simulink model "circuitosLogicos"  (R2014a)
settings: Solver=ode45  StartTime=0.0  StopTime=inf  MaxStep=0.01  RelTol=1e-3
settings Model: Creator=gbtom  LastModifiedBy=gbtom

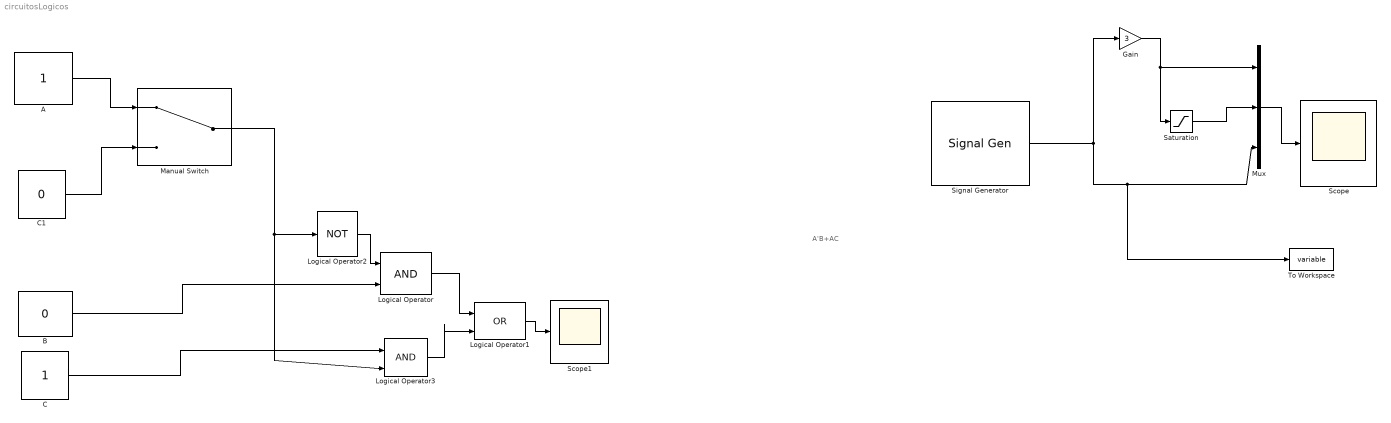
== system circuitosLogicos ==
  note: A'B+AC
  A : Constant
  B : Constant  Value=0
  C : Constant
  C1 : Constant  Value=0
  Gain : Gain  Gain=3
  Logical Operator : Logic  IconShape=distinctive  AllPortsSameDT=off  OutDataTypeStr=boolean
  Logical Operator1 : Logic  Operator=OR  IconShape=distinctive  AllPortsSameDT=off  OutDataTypeStr=boolean
  Logical Operator2 : Logic  Operator=NOT  IconShape=distinctive  AllPortsSameDT=off  OutDataTypeStr=boolean
  Logical Operator3 : Logic  IconShape=distinctive  AllPortsSameDT=off  OutDataTypeStr=boolean
  Manual Switch : ManualSwitch
  Mux : Mux  Inputs=3
  Saturation : Saturate  UpperLimit=10  LowerLimit=-10
  Scope : Scope
      settings: YMin=-15  YMax=15
  Scope1 : Scope
  Signal Generator : SignalGenerator  Amplitude=5
  To Workspace : ToWorkspace  VariableName=variable  SaveFormat=Timeseries  SampleTime=-1
  wires:
  Signal Generator/1 -> To Workspace/1, Mux/3, Gain/1
  Mux/1 -> Scope/1
  Saturation/1 -> Mux/2
  Gain/1 -> Saturation/1, Mux/1
  Logical Operator2/1 -> Logical Operator/1
  Logical Operator3/1 -> Logical Operator1/2
  Logical Operator/1 -> Logical Operator1/1
  Logical Operator1/1 -> Scope1/1
  B/1 -> Logical Operator/2
  C/1 -> Logical Operator3/1
  C1/1 -> Manual Switch/2
  A/1 -> Manual Switch/1
  Manual Switch/1 -> Logical Operator3/2, Logical Operator2/1
